simulink model "Open_Loop_shift_notol_initial"  (R2015a)
settings: Solver=ode3  StartTime=0.0  StopTime=200  FixedStep=0.01  MaxStep=0.01  RelTol=1e-3
values from neighbouring files (symbols this model uses):
  H0 = Periodic_Solution(1,4)+sqrt(tol)*cos(Phi)    [Error_check.m]
  n0 = rand    [Error_check.m]
  Periodic_Solution = Periodic_Solution(N:end,:)    [Error_check.m]
  Sleep0 = Periodic_Solution(1,6)    [Error_check.m]
  x0 = Periodic_Solution(1,2)+sqrt(tol)*sin(Phi)*cos(Theta)    [Error_check.m]
  xc0 = Periodic_Solution(1,3)+sqrt(tol)*sin(Phi)*sin(Theta)    [Error_check.m]
settings Model: Creator=wangf7  LastModifiedBy=Jiawei Yin
settings OptimizationCC: ExpressionDepthLimit=2147483647
settings DebuggingCC: AlgebraicLoopMsg=none  ArtificialAlgebraicLoopMsg=none  UnderspecifiedInitializationDetection=Classic  MergeDetectMultiDrivingBlocksExec=none  SolverPrmCheckMsg=warning  StateNameClashWarn=warning

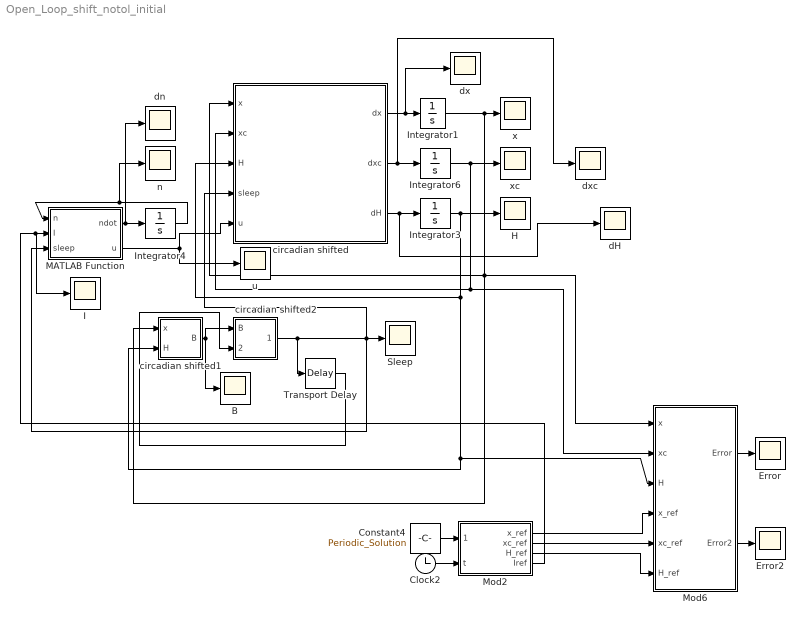
== system Open_Loop_shift_notol_initial ==
  B : Scope
      settings: TimeRange=auto  MaxDataPoints=5000  SaveName=B  YMin=-10  YMax=10  SampleTime=-1  DataFormat=Array
  Clock2 : Clock
  Constant4 : Constant  Value=Periodic_Solution
  Error : Scope
      settings: TimeRange=auto  MaxDataPoints=5000  SaveName=Error  YMin=-0.00116  YMax=0.01124  SampleTime=-1  DataFormat=Array
  Error2 : Scope
      settings: TimeRange=auto  MaxDataPoints=5000  SaveName=Error2  YMin=-0.12348  YMax=0.1213  SampleTime=-1  DataFormat=Array
  H : Scope
      settings: TimeRange=auto  MaxDataPoints=5000  SaveName=H  YMin=0.08394  YMax=0.57854  SampleTime=-1  DataFormat=Array
  I : Scope
      settings: TimeRange=auto  MaxDataPoints=5000  SaveName=I  YMin=-1250.00000  YMax=11250.00000  SampleTime=-1  DataFormat=Array
  Integrator1 : Integrator  InitialCondition=x0
  Integrator3 : Integrator  InitialCondition=H0
  Integrator4 : Integrator  InitialCondition=n0
  Integrator6 : Integrator  InitialCondition=xc0
  MATLAB Function : MATLAB Function  TreatAsAtomicUnit=on
      settings: PermitHierarchicalResolution=ParametersOnly
  Mod2 : MATLAB Function  TreatAsAtomicUnit=on
      settings: PermitHierarchicalResolution=ParametersOnly
  Mod6 : MATLAB Function  TreatAsAtomicUnit=on
      settings: PermitHierarchicalResolution=ParametersOnly
  Sleep : Scope
      settings: TimeRange=auto  MaxDataPoints=5000  SaveName=Sleep  YMin=-0.125  YMax=1.125  SampleTime=-1  DataFormat=Array
  Transport Delay : TransportDelay  DelayTime=.01  InitialOutput=Sleep0
  circadian shifted : MATLAB Function  TreatAsAtomicUnit=on
      settings: PermitHierarchicalResolution=ParametersOnly
  circadian shifted1 : MATLAB Function  TreatAsAtomicUnit=on
      settings: PermitHierarchicalResolution=ParametersOnly
  circadian shifted2 : MATLAB Function  TreatAsAtomicUnit=on
      settings: PermitHierarchicalResolution=ParametersOnly
  dH : Scope
      settings: TimeRange=auto  MaxDataPoints=5000  SaveName=dH  YMin=0.03966  YMax=0.05966  SampleTime=-1  DataFormat=Array
  dn : Scope
      settings: TimeRange=auto  MaxDataPoints=5000  SaveName=dn  YMin=-10  YMax=10  SampleTime=-1  DataFormat=Array
  dx : Scope
      settings: TimeRange=auto  MaxDataPoints=5000  SaveName=dx  YMin=-10  YMax=10  SampleTime=-1  DataFormat=Array
  dxc : Scope
      settings: TimeRange=auto  MaxDataPoints=5000  SaveName=dxc  YMin=-10  YMax=10  SampleTime=-1  DataFormat=Array
  n : Scope
      settings: TimeRange=auto  MaxDataPoints=5000  SaveName=n  YMin=-10  YMax=10  SampleTime=-1  DataFormat=Array
  u : Scope
      settings: TimeRange=auto  MaxDataPoints=5000  SaveName=u  YMin=-0.12852  YMax=1.15668  SampleTime=-1  DataFormat=Array
  x : Scope
      settings: TimeRange=auto  MaxDataPoints=5000  SaveName=x  YMin=-0.56951  YMax=1.25946  SampleTime=-1  DataFormat=Array
  xc : Scope
      settings: TimeRange=auto  MaxDataPoints=5000  SaveName=xc  YMin=-1.29593  YMax=1.31086  SampleTime=-1  DataFormat=Array
  wires:
  circadian shifted/1(dx) -> Integrator1/1, dx/1
  Integrator1/1 -> circadian shifted1/1(x), Mod6/1(x), circadian shifted/1(x), x/1
  Integrator6/1 -> Mod6/2(xc), circadian shifted/2(xc), xc/1
  Constant4/1 -> Mod2/1(Periodic_Solution)
  Clock2/1 -> Mod2/2(t)
  Mod6/1(Error) -> Error/1
  Mod2/3(H_ref) -> Mod6/6(H_ref)
  circadian shifted/2(dxc) -> dxc/1, Integrator6/1
  Integrator3/1 -> circadian shifted1/2(H), Mod6/3(H), circadian shifted/3(H), H/1
  Mod2/1(x_ref) -> Mod6/4(x_ref)
  Mod2/2(xc_ref) -> Mod6/5(xc_ref)
  circadian shifted/3(dH) -> dH/1, Integrator3/1
  Mod2/4(Iref) -> I/1, MATLAB Function/2(I)
  MATLAB Function/2(u) -> circadian shifted/5(u), u/1
  MATLAB Function/1(ndot) -> dn/1, Integrator4/1
  Integrator4/1 -> n/1, MATLAB Function/1(n)
  circadian shifted1/1(B) -> circadian shifted2/1(B), B/1
  circadian shifted2/1(Sleep) -> Transport Delay/1, MATLAB Function/3(sleep), Sleep/1, circadian shifted/4(sleep)
  Transport Delay/1 -> circadian shifted2/2(Sleep0)
  Mod6/2(Error2) -> Error2/1

== matlab function Open_Loop_shift_notol_initial/circadian shifted1 ==
  data: x input; H input; B output
function B = fcn(x,H)
%#eml
B=H-0.1333*x;

== matlab function Open_Loop_shift_notol_initial/circadian shifted2 ==
  data: B input; Sleep0 input; Sleep output
function Sleep = fcn(B,Sleep0)
%#eml
Sleep=round(Sleep0);
if B<=0.17
    Sleep=0;
end
if B>=0.67
    Sleep=1;
end

== matlab function Open_Loop_shift_notol_initial/MATLAB Function ==
  data: n input; I input; ndot output; u output; sleep input
function [ndot,u] = fcn(n,I,sleep)
G=33.75;
alpha0=0.05;
beta=0.0075;
I0=9500;

alpha=alpha0*(I/I0)^0.5;
u=G*alpha*(1-n)*(1-sleep);
ndot=60*[alpha*(1-n)*(1-sleep)-beta*n];

== matlab function Open_Loop_shift_notol_initial/circadian shifted ==
  data: x input; xc input; H input; sleep input; u input; dx output; dxc output; dH output
function [dx,dxc,dH] = fcn(x,xc,H,sleep,u)
%#eml

tr=18.2;
td=4.2;

q = 1/3;
taux = 24.2;
k = 0.55;
mu=0.13;

B = u*(1-0.4*x)*(1-0.4*xc)*(1-sleep);

dx = (pi/12)*(xc + B  + mu*(1/3*x + 4/3*x^3 - 256/105*x^7));
dxc = (pi/12)*(q*B *xc - (24/(taux*0.99729))^2*x - k*B*x);
dH = (1-sleep)*(1-H)/tr-(H*sleep)/td;

== matlab function Open_Loop_shift_notol_initial/Mod2 ==
  data: Periodic_Solution input; x_ref output; xc_ref output; t input; H_ref output; Iref output
function [x_ref,xc_ref,H_ref,Iref] = fcn(Periodic_Solution,t)
%#codegen
x_ref=interp1q(Periodic_Solution(:,1),Periodic_Solution(:,2),t);
xc_ref=interp1q(Periodic_Solution(:,1),Periodic_Solution(:,3),t);
H_ref=interp1q(Periodic_Solution(:,1),Periodic_Solution(:,4),t);
Iref=interp1q(Periodic_Solution(:,1),Periodic_Solution(:,5),t);

== matlab function Open_Loop_shift_notol_initial/Mod6 ==
  data: Error output; x input; xc input; H input; x_ref input; xc_ref input; H_ref input; Error2 output
function [Error,Error2]  = fcn(x,xc,H,x_ref,xc_ref,H_ref)
%#codegen
Error=(H-H_ref)^2+(x-x_ref)^2+(xc-xc_ref)^2;
Error2=[x-x_ref;xc-xc_ref;H-H_ref];
